simulink model "undirect_graph_compare_pioneer"  (R2020a)
settings: Solver=FixedStepAuto  StartTime=0.0  StopTime=10.0  FixedStep=0.0001  RelTol=1e-3
settings Model: Creator=WangQipeng  LastModifiedBy=WangQipeng

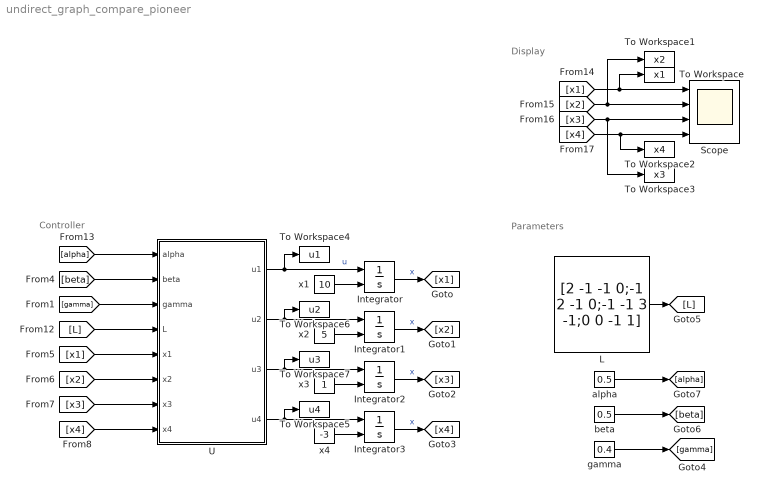
== system undirect_graph_compare_pioneer ==
  note: Controller
  note: Display
  note: Parameters
  Integrator{,1..3} (4 alike) : Integrator  InitialConditionSource=external  InitialCondition=1
  L : Constant  Value=[2 -1 -1 0;-1 2 -1 0;-1 -1 3 -1;0 0 -1 1]
  Scope : Scope  NumInputPorts=4
  To Workspace : ToWorkspace  VariableName=x1  SaveFormat=Timeseries  SampleTime=-1
  To Workspace1 : ToWorkspace  VariableName=x2  SaveFormat=Timeseries  SampleTime=-1
  To Workspace2 : ToWorkspace  VariableName=x4  SaveFormat=Timeseries  SampleTime=-1
  To Workspace3 : ToWorkspace  VariableName=x3  SaveFormat=Timeseries  SampleTime=-1
  To Workspace4 : ToWorkspace  VariableName=u1  SaveFormat=Timeseries  SampleTime=-1
  To Workspace5 : ToWorkspace  VariableName=u4  SaveFormat=Timeseries  SampleTime=-1
  To Workspace6 : ToWorkspace  VariableName=u2  SaveFormat=Timeseries  SampleTime=-1
  To Workspace7 : ToWorkspace  VariableName=u3  SaveFormat=Timeseries  SampleTime=-1
  U : MATLAB Function  TreatAsAtomicUnit=on
  alpha : Constant  Value=0.5
  beta : Constant  Value=0.5
  gamma : Constant  Value=0.4
  x1 : Constant  Value=10
  x2 : Constant  Value=5
  x3 : Constant
  x4 : Constant  Value=-3
  wires:
  U/1(u1) -> To Workspace4/1, Integrator/1  "u"
  U/2(u2) -> To Workspace6/1, Integrator1/1
  U/3(u3) -> To Workspace7/1, Integrator2/1
  U/4(u4) -> To Workspace5/1, Integrator3/1
  Integrator/1 -> [x1]  "x"
  Integrator1/1 -> [x2]  "x"
  Integrator2/1 -> [x3]  "x"
  Integrator3/1 -> [x4]  "x"
  [beta] -> U/2(beta)
  [x3] -> U/7(x3)
  [x4] -> U/8(x4)
  [x1] -> U/5(x1)
  [x2] -> U/6(x2)
  L/1 -> [L]
  beta/1 -> [beta]
  alpha/1 -> [alpha]
  [L] -> U/4(L)
  [alpha] -> U/1(alpha)
  x1/1 -> Integrator/2
  x2/1 -> Integrator1/2
  x3/1 -> Integrator2/2
  x4/1 -> Integrator3/2
  [x1] -> To Workspace/1, Scope/1
  [x2] -> Scope/2, To Workspace1/1
  [x3] -> Scope/3, To Workspace3/1
  [x4] -> Scope/4, To Workspace2/1
  gamma/1 -> [gamma]
  [gamma] -> U/3(gamma)

== matlab function undirect_graph_compare_pioneer/U ==
  data: alpha input; u1 output; beta input; gamma input; L input; x1 input; x2 input; x3 input; x4 input; u2 output; u3 output; u4 output
function [u1,u2,u3,u4] = protocol(alpha,beta,gamma,L,x1,x2,x3,x4)
x = [x1;x2;x3;x4];
temp = -L * x;
temp_u1 = temp(1);
temp_u2 = temp(2);
temp_u3 = temp(3);
temp_u4 = temp(4);

u1 = alpha * sign(temp_u1) * abs(temp_u1)^(2-gamma) + beta * sign(temp_u1) * abs(temp_u1)^gamma;
u2 = alpha * sign(temp_u2) * abs(temp_u2)^(2-gamma) + beta * sign(temp_u2) * abs(temp_u2)^gamma;
u3 = alpha * sign(temp_u3) * abs(temp_u3)^(2-gamma) + beta * sign(temp_u3) * abs(temp_u3)^gamma;
u4 = alpha * sign(temp_u4) * abs(temp_u4)^(2-gamma) + beta * sign(temp_u4) * abs(temp_u4)^gamma;
